simulink model "LQR"  (R2023b)
settings: Solver=VariableStepAuto  StartTime=0.0  StopTime=50  RelTol=1e-3
values from neighbouring files (symbols this model uses):
  A = [ -8.8487+(a-b)/5,           -0.0399,                     -5.55+(c+d)/10,               3.5846 ... (first row only)    [LQR_codes.m]    (also in Q2.m)
  B = [0.0564+b/(10+c),                       0.0319 ... (first row only)    [LQR_codes.m]    (also in Q2.m)
  C = [-3.2988,              -2.1932+(10*c+d)/(100+5*a),  0.037,      -0.0109 ... (first row only)    [LQR_codes.m]    (also in Q2.m)
  K_LQR = lqr(A, B, Q2.*Q(i), R)    [LQR_codes.m]    (also in Q2.m = inv(R)*B'*P)
  x0 = [0; 0; 0; 0]    [LQR_codes.m]    (also in Q2.m)
settings Model: Creator=wyton  LastModifiedBy=shipingguo
settings SolverCC: AlgebraicLoopSolver=TrustRegion
settings DataIOCC: SaveState=on
settings OptimizationCC: ReuseModelBlockBuffer=off
settings DebuggingCC: UnconnectedInputMsg=warning  UnconnectedOutputMsg=warning  UnconnectedLineMsg=warning
settings ModelReferenceCC: EnableRefExpFcnMdlSchedulingChecks=on
settings RTWCC: DLArmComputeVersion=19.05

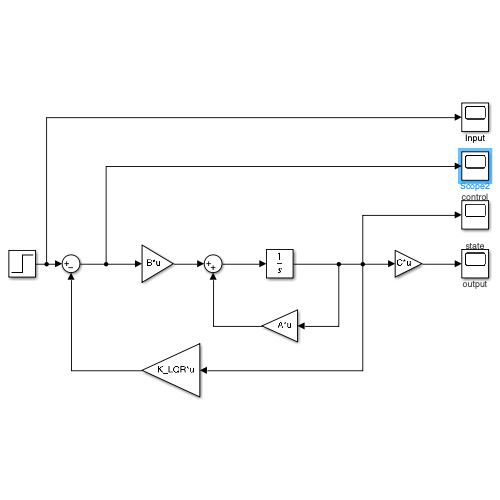
[thumbnail: Simulink's stored preview of the top-level diagram]
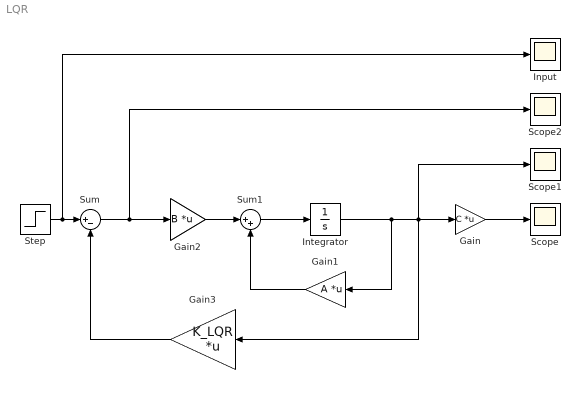
== system LQR ==
  Gain : Gain  Gain=C  Multiplication=Matrix(K*u)
  Gain1 : Gain  Gain=A  Multiplication=Matrix(K*u)
  Gain2 : Gain  Tag=B  Gain=B  Multiplication=Matrix(K*u)
  Gain3 : Gain  Gain=K_LQR  Multiplication=Matrix(K*u)
  Input : Scope
  Integrator : Integrator  InitialCondition=x0
  Scope : Scope
      settings: AttributesFormatString=output
  Scope1 : Scope
      settings: AttributesFormatString=state
  Scope2 : Scope
      settings: AttributesFormatString=control
  Step : Step  Time=0  Before=[0,0]  After=[0,0]  SampleTime=0
  Sum : Sum  Inputs=|+-
  Sum1 : Sum  Inputs=|++
  wires:
  Step/1 -> Input/1, Sum/1
  Sum/1 -> Scope2/1, Gain2/1
  Sum1/1 -> Integrator/1
  Gain2/1 -> Sum1/1
  Integrator/1 -> Gain1/1, Gain3/1, Gain/1, Scope1/1
  Gain1/1 -> Sum1/2
  Gain/1 -> Scope/1
  Gain3/1 -> Sum/2
